simulink model "single_cmg_practice"  (R2023b)
settings: Solver=ode4  StartTime=0.0  StopTime=1000  FixedStep=0.001  RelTol=1e-3
undefined symbols (not defined in the file): As, Cube_L, F_vec, I_rw1, M_c, M_rw, sat, THR_Force, THR_Pos, torque_ext, X, Y, Z
libraries: sm_lib x391, nesl_utility x251, simulink_extras x103, sharedtransform x53, aerolibutil x30, sharedutil x13, simulink x12
(part 13 of 14)

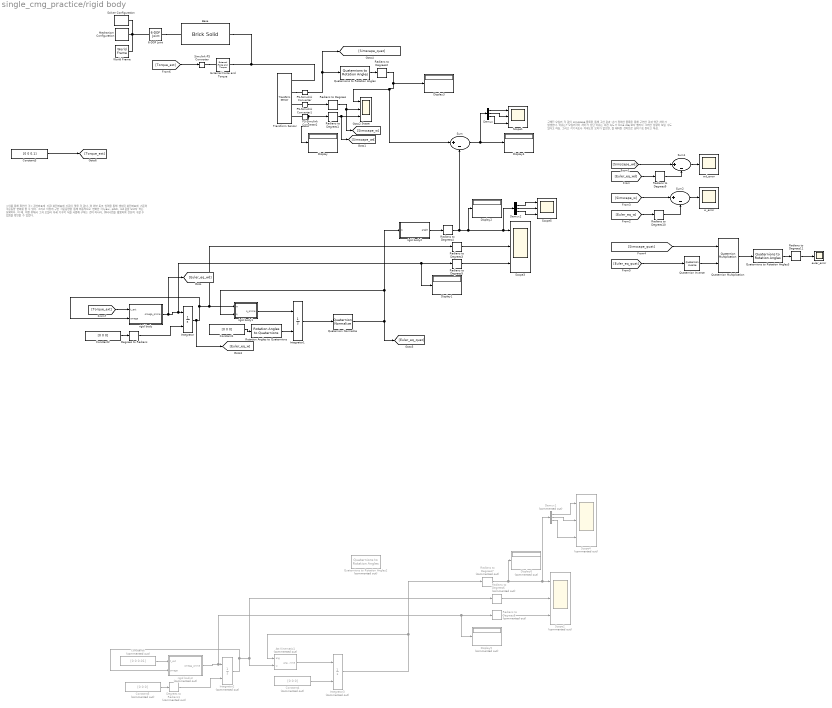
== system single_cmg_practice/rigid body ==
  note: 구해진 오일러 각 값이
      | simscape 블록을 통해 구한 값과 내가 정의한 블록을 통해 구현한 값과
      | 약간 차이가 발생한다.
      | 이유는?
      | 오일러각이 차이가 났던 이유는 회전 속도가 time step보다 빨라서 그러한 상황이 보일 수도 있다고 하심.
      | 그리고 각가속도나 각속도의 오차가 없으면, 잘 제어된 것이므로 넘어가도 된다고 하심.
  note: <이를 통해 확인한 것>
      | 관선좌표계 기준(회전좌표계 기준이 맞을 것 같다.)의 외부 토크 입력을 통해
      | 생성된 회전좌표계 기준의 각운동량 변화를 볼 수 있다.
      |
      | 그리고 이렇게 구한 각운동량을 통해
      | 최종적으로 변화한 각(yaw, pitch, roll)값을 보고자 하는 상황이다.
      | 이 때, 이를 위해서 그저 오일러 자세 기구학 식을 사용해 구하는 것이 아니라,
      | 쿼터니언을 활용하여 간단히 구할 수 있음을 확인할 수 있었다.
  6-DOF Joint : sm_lib/Joints/6-DOF Joint  JointMode=Normal  SenseConstraintForce=off  SenseConstraintForceX=off  SenseConstraintForceY=off  SenseConstraintForceZ=off  SenseConstraintTorque=off  SenseConstraintTorqueX=off  SenseConstraintTorqueY=off  SenseConstraintTorqueZ=off  SenseTotalForce=off  SenseTotalForceX=off  SenseTotalForceY=off  SenseTotalForceZ=off  SenseTotalTorque=off  SenseTotalTorqueX=off  SenseTotalTorqueY=off  SenseTotalTorqueZ=off  CompositeWrenchDir=FollowerOnBase  CompositeWrenchFrame=BaseFrame  PxEquilibriumPosition=0  PxEquilibriumPositionUnits=m  PxSpringStiffness=0  PxSpringStiffnessUnits=N/m  PxDampingCoefficient=0  PxDampingCoefficientUnits=N/(m/s)  PxTorqueActuationMode=NoTorque  PxMotionActuationMode=ComputedMotion  PxSensePosition=off  PxSenseVelocity=off  PxSenseAcceleration=off  PxSenseTorqueForce=off  PxSenseLowerLimitTorqueForce=off  PxSenseUpperLimitTorqueForce=off  PxLowerLimitSpecify=off  PxLowerLimitBound=-1  PxLowerLimitBoundUnits=m  PxLowerLimitStiffness=1e6  PxLowerLimitStiffnessUnits=N/m  PxLowerLimitDamping=1e3  PxLowerLimitDampingUnits=N/(m/s)  PxLowerLimitTransitionRegionWidth=1e-4  PxLowerLimitTransitionRegionWidthUnits=m  PxUpperLimitSpecify=off  PxUpperLimitBound=1  PxUpperLimitBoundUnits=m  PxUpperLimitStiffness=1e6  PxUpperLimitStiffnessUnits=N/m  PxUpperLimitDamping=1e3  PxUpperLimitDampingUnits=N/(m/s)  PxUpperLimitTransitionRegionWidth=1e-4  PxUpperLimitTransitionRegionWidthUnits=m  PxPositionTargetSpecify=off  PxPositionTargetPriority=High  PxPositionTargetValue=0  PxPositionTargetValueUnits=m  PxVelocityTargetSpecify=off  PxVelocityTargetPriority=High  PxVelocityTargetValue=0  PxVelocityTargetValueUnits=m/s  PyEquilibriumPosition=0  PyEquilibriumPositionUnits=m  PySpringStiffness=0  PySpringStiffnessUnits=N/m  PyDampingCoefficient=0  PyDampingCoefficientUnits=N/(m/s)  PyTorqueActuationMode=NoTorque  PyMotionActuationMode=ComputedMotion  PySensePosition=off  PySenseVelocity=off  PySenseAcceleration=off  PySenseTorqueForce=off  PySenseLowerLimitTorqueForce=off  PySenseUpperLimitTorqueForce=off  PyLowerLimitSpecify=off  PyLowerLimitBound=-1  PyLowerLimitBoundUnits=m  PyLowerLimitStiffness=1e6  PyLowerLimitStiffnessUnits=N/m  PyLowerLimitDamping=1e3  PyLowerLimitDampingUnits=N/(m/s)  PyLowerLimitTransitionRegionWidth=1e-4  PyLowerLimitTransitionRegionWidthUnits=m  PyUpperLimitSpecify=off  PyUpperLimitBound=1  PyUpperLimitBoundUnits=m  PyUpperLimitStiffness=1e6  PyUpperLimitStiffnessUnits=N/m  PyUpperLimitDamping=1e3  PyUpperLimitDampingUnits=N/(m/s)  PyUpperLimitTransitionRegionWidth=1e-4  PyUpperLimitTransitionRegionWidthUnits=m  PyPositionTargetSpecify=off  PyPositionTargetPriority=High  PyPositionTargetValue=0  PyPositionTargetValueUnits=m  PyVelocityTargetSpecify=off  PyVelocityTargetPriority=High  PyVelocityTargetValue=0  PyVelocityTargetValueUnits=m/s  PzEquilibriumPosition=0  PzEquilibriumPositionUnits=m  PzSpringStiffness=0  PzSpringStiffnessUnits=N/m  PzDampingCoefficient=0  PzDampingCoefficientUnits=N/(m/s)  PzTorqueActuationMode=NoTorque  PzMotionActuationMode=ComputedMotion  PzSensePosition=off  PzSenseVelocity=off  PzSenseAcceleration=off  PzSenseTorqueForce=off  PzSenseLowerLimitTorqueForce=off  PzSenseUpperLimitTorqueForce=off  PzLowerLimitSpecify=off  PzLowerLimitBound=-1  PzLowerLimitBoundUnits=m  PzLowerLimitStiffness=1e6  PzLowerLimitStiffnessUnits=N/m  PzLowerLimitDamping=1e3  PzLowerLimitDampingUnits=N/(m/s)  PzLowerLimitTransitionRegionWidth=1e-4  PzLowerLimitTransitionRegionWidthUnits=m  PzUpperLimitSpecify=off  PzUpperLimitBound=1  PzUpperLimitBoundUnits=m  PzUpperLimitStiffness=1e6  PzUpperLimitStiffnessUnits=N/m  PzUpperLimitDamping=1e3  PzUpperLimitDampingUnits=N/(m/s)  PzUpperLimitTransitionRegionWidth=1e-4  PzUpperLimitTransitionRegionWidthUnits=m  PzPositionTargetSpecify=off  PzPositionTargetPriority=High  PzPositionTargetValue=0  PzPositionTargetValueUnits=m  PzVelocityTargetSpecify=off  PzVelocityTargetPriority=High  PzVelocityTargetValue=0  PzVelocityTargetValueUnits=m/s  SphEqPosRotationMethod=None  SphEqPosRotationAngleUnits=deg  SphEqPosRotationStandardAxis=+Z  SphEqPosRotationAngle=0.0  SphEqPosRotationArbitraryAxis=[0 0 1]  SphEqPosFollAlignAxisA=+X  SphEqPosBaseAlignAxisA=+Y  SphEqPosFollAlignAxisB=+Y  SphEqPosBaseAlignAxisB=+Z  SphEqPosRotationSequenceAxes=FollowerAxes  SphEqPosRotationSequence=XYX  SphEqPosRotationSequenceAngles=[0 0 0]  SphEqPosRotationSequenceAnglesUnits=deg  SphEqPosRotationMatrix=[1 0 0; 0 1 0; 0 0 1]  SphEqPosQuaternion=[1 0 0 0]  SphSpringStiffness=0  SphSpringStiffnessUnits=N*m/deg  SphDampingCoefficient=0  SphDampingCoefficientUnits=N*m/(deg/s)  SphActuateTorqueX=off  SphActuateTorqueY=off  SphActuateTorqueZ=off  SphActuateTorque=off  SphTorqueActuationMode=NoTorque  SphMotionActuationMode=ComputedMotion  SphActuationFrame=BaseFrame  SphSensePosition=off  SphSenseVelocityX=off  SphSenseVelocityY=off  SphSenseVelocityZ=off  SphSenseVelocity=off  SphSenseAccelerationX=off  SphSenseAccelerationY=off  SphSenseAccelerationZ=off  SphSenseAcceleration=off  SphSenseTorqueX=off  SphSenseTorqueY=off  SphSenseTorqueZ=off  SphSenseTorqueForce=off  SphSenseLowerLimitTorqueMag=off  SphSenseUpperLimitTorqueMag=off  SphSensingFrame=BaseFrame  SphLowerLimitSpecify=off  SphLowerLimitBound=15  SphLowerLimitBoundUnits=deg  SphLowerLimitStiffness=1e4  SphLowerLimitStiffnessUnits=N*m/deg  SphLowerLimitDamping=10  SphLowerLimitDampingUnits=N*m/(deg/s)  SphLowerLimitTransitionRegionWidth=0.1  SphLowerLimitTransitionRegionWidthUnits=deg  SphUpperLimitSpecify=off  SphUpperLimitBound=45  SphUpperLimitBoundUnits=deg  SphUpperLimitStiffness=1e4  SphUpperLimitStiffnessUnits=N*m/deg  SphUpperLimitDamping=10  SphUpperLimitDampingUnits=N*m/(deg/s)  SphUpperLimitTransitionRegionWidth=0.1  SphUpperLimitTransitionRegionWidthUnits=deg  SphPositionTargetRotationMethod=None  SphPositionTargetRotationAngleUnits=deg  SphPositionTargetRotationStandardAxis=+Z  SphPositionTargetRotationAngle=0.0  SphPositionTargetRotationArbitraryAxis=[0 0 1]  SphPositionTargetFollAlignAxisA=+X  SphPositionTargetBaseAlignAxisA=+Y  SphPositionTargetFollAlignAxisB=+Y  SphPositionTargetBaseAlignAxisB=+Z  SphPositionTargetRotationSequenceAxes=FollowerAxes  SphPositionTargetRotationSequence=XYX  SphPositionTargetRotationSequenceAngles=[0 0 0]  SphPositionTargetRotationSequenceAnglesUnits=deg  SphPositionTargetRotationMatrix=[1 0 0; 0 1 0; 0 0 1]  SphPositionTargetQuaternion=[1 0 0 0]  SphPositionTargetSpecify=off  SphPositionTargetPriority=High  SphVelocityTargetValue=[0 0 0]  SphVelocityTargetValueUnits=deg/s  SphVelocityTargetSpecify=off  SphVelocityTargetPriority=High  SphVelocityTargetInFollowerFrame=on
  Att Kinematic1 : MATLAB Function  Commented=on  TreatAsAtomicUnit=on
  Base : sm_lib/Body Elements/Brick Solid  GraphicAmbientColor=[0.15 0.15 0.15 1.0]  BasedOnType=Mass  BrickDimensions=[0.3 0.3 0.3]  BrickDimensionsUnits=m  CenterOfMass=[0 0 0]  CenterOfMassUnits=m  GraphicDiffuseColor=[0.0 0.8 0.8]  Density=1000  DensityUnits=kg/m^3  DoExposeReferenceFrame=on  GraphicEmissiveColor=[0.0 0.0 0.0 1.0]  ExportEntireGeometry=off  SerializedFrames=<Frames><Frame><Id>Frame1</Id><Value><Name>CM_F</Name><Origin><Source>CenterOfMassFrame</Source><FeatureName></FeatureName></Origin><PrimaryAxis><DefinedDirection>+Z</DefinedDirection><Source>ReferenceFrame</Source><SourceDirection>+Z</SourceDirection><FeatureName></FeatureName></PrimaryAxis><SecondaryAxis><DefinedDirection>+X</DefinedDirection><Source>ReferenceFrame</Source><SourceDirection>+X</SourceDirection><FeatureName></FeatureName></SecondaryAxis></Value></Frame></Frames>  MarkerShape=Sphere  MarkerSize=10  GraphicType=FromGeometry  InertiaType=CalculateFromGeometry  Mass=1  MassUnits=kg  MomentsOfInertia=[1 1 1]  MomentsOfInertiaUnits=kg*m^2  GraphicOpacity=1  ProductsOfInertia=[0 0 0]  ProductsOfInertiaUnits=kg*m^2  GraphicShininess=75  GraphicSpecularColor=[0.5 0.5 0.5 1.0]  GraphicVisPropType=SimpleVisualProperties
  Constant1 : Constant  Value=[0 0 0]
  Constant2 : Constant  Value=[0 0 0]
  Constant3 : Constant  Value=[0 0 0.1]
  Constant4 : Constant  Commented=on  Value=[0 0 0]
  Constant5 : Constant  Commented=on  Value=[0 0 0]
  Constant6 : Constant  Commented=on  Value=[0 0 0.01]
  Degrees to Radians : simulink_extras/Transformations/Degrees to Radians
  Degrees to Radians1 : simulink_extras/Transformations/Degrees to Radians  Commented=on
  Demux : Demux  Outputs=3
  Demux1 : Demux  Commented=on  Outputs=3
  Demux2 : Demux  Outputs=3
  Display{,1..4} (5 alike) : Display
  Display5 : Display  Commented=on
  Display6 : Display  Commented=on
  External Force and Torque : sm_lib/Forces and Torques/External Force and Torque  ForceResolutionFrame=AttachedFrame  EnableForceX=off  EnableForceY=off  EnableForceZ=off  EnableForce=off  TorqueResolutionFrame=AttachedFrame  EnableTorqueX=off  EnableTorqueY=off  EnableTorqueZ=off  EnableTorque=on
  Integrator : Integrator  InitialConditionSource=external
  Integrator1 : Integrator  InitialConditionSource=external
  Integrator2 : Integrator  Commented=on  InitialConditionSource=external
  Integrator3 : Integrator  Commented=on  InitialConditionSource=external
  Mechanism Configuration : sm_lib/Utilities/Mechanism Configuration  UniformGravity=None  GravityVector=[0 0 -9.80665]  GravityVectorUnits=m/s^2  LinearizationDelta=0.001  JointModeTransitionNonlinearIterations=2
  PS-Simulink Converter : nesl_utility/PS-Simulink Converter  PhysicalDomain=network_engine_domain  SubClassName=ps_output  LeftPortType=input  RightPortType=output  PseudoPeriodic=off  Frequencies=[]  VectorFormat=inherit  Unit=inherit  AffineConversion=off
  PS-Simulink Converter1 : nesl_utility/PS-Simulink Converter  PhysicalDomain=network_engine_domain  SubClassName=ps_output  LeftPortType=input  RightPortType=output  PseudoPeriodic=off  Frequencies=[]  VectorFormat=inherit  Unit=inherit  AffineConversion=off
  PS-Simulink Converter2 : nesl_utility/PS-Simulink Converter  PhysicalDomain=network_engine_domain  SubClassName=ps_output  LeftPortType=input  RightPortType=output  PseudoPeriodic=off  Frequencies=[]  VectorFormat=inherit  Unit=inherit  AffineConversion=off
  Quaternion Inverse : aerolibutil/Quaternion Inverse
  Quaternion Multiplication : aerolibutil/Quaternion Multiplication
  Quaternion Normalize : sharedutil/Quaternion Normalize  aMode=aMode
  Quaternions to Rotation Angles : sharedtransform/Quaternions to Rotation Angles  rotationOrder=ZYX  aMode=aMode
  Quaternions to Rotation Angles2 : sharedtransform/Quaternions to Rotation Angles  Commented=on  rotationOrder=ZYX  aMode=aMode
  Quaternions to Rotation Angles3 : sharedtransform/Quaternions to Rotation Angles  rotationOrder=ZYX  aMode=aMode
  Radians to Degrees{,1..5,9..11} (9 alike) : simulink_extras/Transformations/Radians to Degrees
  Radians to Degrees6 : simulink_extras/Transformations/Radians to Degrees  Commented=on
  Radians to Degrees7 : simulink_extras/Transformations/Radians to Degrees  Commented=on
  Radians to Degrees8 : simulink_extras/Transformations/Radians to Degrees  Commented=on
  Rotation Angles to Quaternions : sharedtransform/Rotation Angles to Quaternions  rotationOrder=ZYX  aMode=aMode
  Scope{,1,3,5} (4 alike) : Scope  NumInputPorts=3
  Scope2 : Scope  Commented=on  NumInputPorts=3
  Scope4 : Scope  Commented=on  NumInputPorts=3
  Simulink-PS Converter : nesl_utility/Simulink-PS Converter  PhysicalDomain=network_engine_domain  SubClassName=ps_input  LeftPortType=input  RightPortType=output  PseudoPeriodic=off  Frequencies=[]  NoiseDistribution=none  NoiseParameters=[]  Unit=1  AffineConversion=off  FilteringAndDerivatives=provide  SimscapeFilterOrder=1  InputFilterTimeConstant=0.001  UdotUserProvided=0
  Solver Configuration : nesl_utility/Solver Configuration  PhysicalDomain=network_engine_domain  SubClassName=solver  LeftPortType=input  RightPortType=generic  Tones=[]  Harmonics=[]  SimulateNoise=off  Profile=off  UseLocalSampling=off  EnableSwitchedLinearOptims=on  FrequencyDomain=off  UseCCode=off  RelTol=0.001  AbsTol=0.001  MinStep=1e-09  ToWorkspace=off  RevertToSquareIcSolve=off  NumHomotopyIterations=100  PhasorMode=off  PhasorModeNumHarmonics=1  ConsistencySolver=NEWTON_XTOL_AFTER_FTOL  IndexReductionMethod=DerivativeReplacement  DoDC=off  ResidualTolerance=1e-09  ConsistencyTolSource=GLOBAL  ConsistencyAbsTol=0.001  ConsistencyRelTol=0.001  ConsistencyTolFactor=0.001  UseLocalSolver=off  LocalSolverChoice=NE_BACKWARD_EULER_ADVANCER  ResolveIndetEquations=on  FunctionEvalNumThread=1  LocalSolverSampleTime=0.001  DoFixedCost=off  MaxNonlinIter=3  MaxModeIter=2  ComputeImpulses=off  ImpulseIterations=2  LinearAlgebra=auto  LinearAlgebraNumThread=0  EquationFormulation=NE_TIME_EF  DelaysMemoryBudget=1024  AutomaticFiltering=on  FilteringTimeConstant=0.001  PartitionStorageMethod=AS_NEEDED  PartitionMemoryBudget=1024  PartitionMethod=ROBUST  MultibodyUseLocalSolver=off  MultibodyLocalSolverChoice=ODE1  MultibodyLocalSolverSampleTime=0.001
  Sum : Sum  Inputs=|+-
  Sum1 : Sum  Inputs=|+-
  Sum2 : Sum  Inputs=|+-
  Transform Sensor : sm_lib/Frames and Transforms/Transform Sensor  MeasurementFrame=World  RotationSequence=ZYX  SenseAngle=off  SenseAxis=off  SenseQ=on  SenseR=off  SenseRotationSequence=off  SenseOmegaX=off  SenseOmegaY=off  SenseOmegaZ=off  SenseOmega=on  SenseQDot=off  SenseRDot=off  SenseRotationSequenceDot=off  SenseAlphaX=off  SenseAlphaY=off  SenseAlphaZ=off  SenseAlpha=on  SenseQDDot=off  SenseRDDot=off  SenseX=off  SenseY=off  SenseZ=off  SenseXYZ=off  SenseRad=off  SenseAzim=off  SenseDist=off  SenseInc=off  SenseXDot=off  SenseYDot=off  SenseZDot=off  SenseXYZDot=off  SenseRadDot=off  SenseAzimDot=off  SenseDistDot=off  SenseIncDot=off  SenseXDDot=off  SenseYDDot=off  SenseZDDot=off  SenseXYZDDot=off  SenseRadDDot=off  SenseAzimDDot=off  SenseDistDDot=off  SenseIncDDot=off
  World Frame : sm_lib/Frames and Transforms/World Frame
  euler_error : Scope
  rigid body : MATLAB Function  TreatAsAtomicUnit=on
  rigid body1 : MATLAB Function  TreatAsAtomicUnit=on
  rigid body2 : MATLAB Function  TreatAsAtomicUnit=on
  rigid body3 : MATLAB Function  Commented=on  TreatAsAtomicUnit=on
  w_error : Scope
  wd_error : Scope
  wires:
  Radians to Degrees/1 -> [Simscape_w], Scope/2
  Radians to Degrees1/1 -> [Simscape_wd], Scope/3
  PS-Simulink Converter2/1 -> Radians to Degrees1/1, Display/1
  PS-Simulink Converter1/1 -> Radians to Degrees/1
  PS-Simulink Converter/1 -> [Simscape_quat], Quaternions to Rotation Angles/1
  Quaternions to Rotation Angles/1 -> Radians to Degrees2/1
  Quaternion Normalize/1 -> rigid body2/1(q), rigid body1/2(q), [Euler_eq_quat]
  Integrator/1 -> rigid body/2(omega), Radians to Degrees3/1, rigid body1/1(w), [Euler_eq_w]
  Constant1/1 -> Rotation Angles to Quaternions/1
  Rotation Angles to Quaternions/1 -> Integrator1/2
  rigid body1/1(q_prime) -> Integrator1/1
  Integrator1/1 -> Quaternion Normalize/1
  Constant2/1 -> Degrees to Radians/1
  Degrees to Radians/1 -> Integrator/2
  rigid body/1(omega_prime) -> [Euler_eq_wd], Display1/1, Radians to Degrees5/1, Integrator/1
  rigid body2/1(angle) -> Radians to Degrees4/1
  Radians to Degrees3/1 -> Scope3/2
  Radians to Degrees5/1 -> Scope3/3
  Sum/1 -> Demux/1, Display4/1
  Demux/1 -> Scope1/1
  Demux/2 -> Scope1/2
  Demux/3 -> Scope1/3
  Radians to Degrees2/1 -> Sum/1, Scope/1, Display3/1
  Integrator3/1 -> Radians to Degrees7/1, Att Kinematic1/1(ang)
  Radians to Degrees8/1 -> Scope2/3
  Constant4/1 -> Integrator3/2
  rigid body3/1(omega_prime) -> Display5/1, Radians to Degrees8/1, Integrator2/1
  Radians to Degrees6/1 -> Scope2/2
  Radians to Degrees7/1 -> Display6/1, Demux1/1, Scope2/1
  Constant6/1 -> rigid body3/1(t_ext)
  Degrees to Radians1/1 -> Integrator2/2
  Att Kinematic1/1(ang_prime) -> Integrator3/1
  Integrator2/1 -> rigid body3/2(omega), Att Kinematic1/2(w), Radians to Degrees6/1
  Constant5/1 -> Degrees to Radians1/1
  Demux1/2 -> Scope4/2
  Demux1/1 -> Scope4/1
  Demux1/3 -> Scope4/3
  Radians to Degrees4/1 -> Sum/2, Display2/1, Demux2/1, Scope3/1
  Demux2/1 -> Scope5/1
  Demux2/2 -> Scope5/2
  Demux2/3 -> Scope5/3
  Sum1/1 -> wd_error/1
  Sum2/1 -> w_error/1
  [Euler_eq_wd] -> Radians to Degrees9/1
  [Simscape_wd] -> Sum1/1
  Radians to Degrees9/1 -> Sum1/2
  [Euler_eq_w] -> Radians to Degrees10/1
  [Simscape_w] -> Sum2/1
  Radians to Degrees10/1 -> Sum2/2
  [Simscape_quat] -> Quaternion Multiplication/1
  [Euler_eq_quat] -> Quaternion Inverse/1
  Quaternion Inverse/1 -> Quaternion Multiplication/2
  Quaternion Multiplication/1 -> Quaternions to Rotation Angles3/1
  Quaternions to Rotation Angles3/1 -> Radians to Degrees11/1
  Constant3/1 -> [Torque_ext]
  [Torque_ext] -> Simulink-PS Converter/1
  [Torque_ext] -> rigid body/1(t_ext)
  Radians to Degrees11/1 -> euler_error/1
  connections:
  Solver Configuration/RConn1 -- 6-DOF Joint/LConn1 -- Mechanism Configuration/RConn1 -- World Frame/RConn1
  6-DOF Joint/RConn1 -- Base/RConn1
  Base/LConn1 -- External Force and Torque/RConn1 -- Transform Sensor/RConn1
  Transform Sensor/RConn2 -- PS-Simulink Converter/LConn1
  PS-Simulink Converter2/LConn1 -- Transform Sensor/RConn4
  PS-Simulink Converter1/LConn1 -- Transform Sensor/RConn3
  Simulink-PS Converter/RConn1 -- External Force and Torque/LConn1

== system single_cmg_practice/CMG_Gimbal_Angle_Control_Example/Subsystem ==
  angle_cmd : Inport
  angle_mea : Inport  Port=2
  rate_mea : Inport  Port=3
  dt : Inport  Port=4
  Trigger : TriggerPort  TriggerType=either  VariantControl=(inherit)  PortDimensions=1
  Gain : Gain
  Gimbal_Angle_Controller[PID] : MATLAB Function  TreatAsAtomicUnit=on
  t_cmd : Outport
  wires:
  angle_cmd/1 -> Gimbal_Angle_Controller[PID]/1(angle_cmd)
  dt/1 -> Gimbal_Angle_Controller[PID]/4(dt)
  Gimbal_Angle_Controller[PID]/1(t_cmd) -> Gain/1
  angle_mea/1 -> Gimbal_Angle_Controller[PID]/2(angle_mea)
  rate_mea/1 -> Gimbal_Angle_Controller[PID]/3(rate_mea)
  Gain/1 -> t_cmd/1

== matlab function single_cmg_practice/Prac1/rigid body1 ==
  data: w input; q_prime output; q input
function q_prime = fcn(w,q)

F_q = (1/2)*[0 -w(1) -w(2) -w(3);
       w(1) 0 w(3) -w(2);
       w(2) -w(3) 0 w(1);
       w(3) w(2) -w(1) 0];

q_prime = F_q*q;

== matlab function single_cmg_practice/Prac1/rigid body2 ==
  data: angle output; q input
function angle = quat2eulang(q)
% ZYX 회전 가정

% q0 = q(1); q1 = q(2); q2 = q(3); q3 = q(4);
% 
% yaw = atan2(2*(q1*q2 + q0*q3), q0^2+q1^2-q2^2-q3^2);
% 
% s = 2*(q0*q2 - q3*q1);
% s = max(-1, min(1, s));      % clamp
% pitch = asin(s);
% 
% roll = atan2(2*(q2*q3 + q0*q1), q0^2-q1^2-q2^2+q3^2);



% % 'ZYX' 회전에서 DCM을 Body-frame -> 관성좌표계 으로 정의할 때, 각을 구하는 상황.
% % /                cos(psi) cos(theta),                              cos(theta) sin(psi),                   -sin(theta)     \
% % |                                                                                                                         |
% % | cos(psi) sin(phi) sin(theta) - cos(phi) sin(psi), cos(phi) cos(psi) + sin(phi) sin(psi) sin(theta), cos(theta) sin(phi) |
% % |                                                                                                                         |
% % \ sin(phi) sin(psi) + cos(phi) cos(psi) sin(theta), cos(phi) sin(psi) sin(theta) - cos(psi) sin(phi), cos(phi) cos(theta) /
R = quat2DCM(q);
yaw   = atan2(R(1,2), R(1,1));
pitch = -asin(R(1,3));
roll  = atan2(R(2,3), R(3,3));



% angle = [roll, pitch, yaw]';
angle = [yaw, pitch, roll]'; %MATLAB 에서는 [roll, pitch, yaw] 가 아닌 [yaw, pitch, roll] 순으로 값을 반환한다.
% 실제 도움말을 보면, 반환각 벡터에 대해 "Ψ is R1, Θ is R2, and Φ is R3." 으로 나와있는 것을 볼 수 있다.



function R = quat2DCM(q)

q0 = q(1); q1 = q(2); q2 = q(3); q3 = q(4);

%% DCM을 관성좌표계 -> Body-frame 으로 정의할 때의 행렬 
% R = [2*(q0^2 + q1^2)-1, 2*(q1*q2 - q0*q3),2*(q1*q3 + q2*q0);
%      2*(q1*q2 + q0*q3), 2*(q0^2 + q2^2)-1, 2*(q2*q3 - q1*q0);
%      2*(q1*q3 - q2*q0), 2*(q2*q3 + q1*q0), 2*(q0^2 + q3^2)-1];

%% DCM을 Body-frame -> 관성좌표계 으로 정의할 때의 행렬 
R = [q0^2+q1^2-q2^2-q3^2, 2*(q1*q2 + q0*q3), 2*(q1*q3 - q2*q0);
     2*(q1*q2 - q0*q3), q0^2-q1^2+q2^2-q3^2, 2*(q2*q3 + q1*q0);
     2*(q1*q3 + q2*q0), 2*(q2*q3 - q1*q0), q0^2-q1^2-q2^2+q3^2];

end

end

== matlab function single_cmg_practice/Prac1/diff_angle ==
  data: angle_err output; q_err input
function angle_err = calc_diff(q_err)

% normalize
q_err = q_err / norm(q_err);

% safe scalar part
q0 = min(abs(q_err(1)),1);

% angle
angle_err = 2*acos(q0);

end

== matlab function single_cmg_practice/Reaction_Wheel_Simple1/rigid body1 ==
  data: I_rw input; u input; omega_rw_prime output; omega input; omega_rw input
% function omega_rw_prime = fcn(u, omega,omega_rw)
function omega_rw_prime = fcn(I_rw,u, omega,omega_rw)
R=0.015; % Radius([m]) of cylinder(Reaction wheel)
M_rw=0.01; % Mass([kg]) of cylinder(Reaction wheel)
L_rw=0.01; % Length([m]) of cylinder(Reaction wheel)

% % MOI([kg*m^2]) of cylinder(Reaction wheel)
% I_rw=[1/4*M_rw*R^2+1/12*M_rw*L_rw^2 0 0;
%     0 1/4*M_rw*R^2+1/12*M_rw*L_rw^2 0;
%     0 0 1/2*M_rw*R^2];

% omega_rw_prime = inv(I_rw)*(-u - cross(omega,I_rw*omega_rw));
omega_rw_prime = inv(I_rw)*(u - cross(omega,I_rw*omega_rw));
% control intput "u" has same direction with "omega_rw_prime"



% % value1 = inv(I_rw)*(1/2*u - cross(omega,I_rw*omega_rw));
% omega_rw_prime + 3.55271e-15

== matlab function single_cmg_practice/Reaction_Wheel_Simple1/rigid body2 ==
  data: Ib input; t_ext input; omega_prime output; omega input; omega_rw input; omega_rw_prime input
function omega_prime = fcn(Ib, t_ext, omega,omega_rw,omega_rw_prime)
L = [0.3 0.3 0.3]'; %Length([m]) of cube 
M = 10; %Mass([kg]) of cube
% MOI([kg*m^2]) of cube
I = [ 1/12*M*(L(2)^2+L(3)^2) 0 0;
      0 1/12*M*(L(1)^2+L(3)^2) 0;
      0 0 1/12*M*(L(1)^2+L(2)^2)];

R=0.015; % Radius([m]) of cylinder(Reaction wheel)
M_rw=0.01; % Mass([kg]) of cylinder(Reaction wheel)
L_rw=0.01; % Length([m]) of cylinder(Reaction wheel)

% MOI([kg*m^2]) of cylinder(Reaction wheel)
I_rw=[1/4*M_rw*R^2+1/12*M_rw*L_rw^2 0 0;
    0 1/4*M_rw*R^2+1/12*M_rw*L_rw^2 0;
    0 0 1/2*M_rw*R^2];

% Ib=I;


omega_prime = inv(Ib)*(t_ext - I_rw*omega_rw_prime - cross(omega, (Ib*omega) + I_rw*omega_rw));

end

== matlab function single_cmg_practice/Reaction_Wheel_Simple1/deriviation of quaternion2 ==
  data: w input; q_prime output; q input
function q_prime = fcn(w,q)

F_q = (1/2)*[0 -w(1) -w(2) -w(3);
       w(1) 0 w(3) -w(2);
       w(2) -w(3) 0 w(1);
       w(3) w(2) -w(1) 0];

q_prime = F_q*q;

== matlab function single_cmg_practice/Reaction_Wheel_Simple1/quaternion to Euler angle 1 ==
  data: angle output; q input
function angle = quat2eulang(q)
% ZYX 회전 가정

% q0 = q(1); q1 = q(2); q2 = q(3); q3 = q(4);
% 
% yaw = atan2(2*(q1*q2 + q0*q3), q0^2+q1^2-q2^2-q3^2);
% 
% s = 2*(q0*q2 - q3*q1);
% s = max(-1, min(1, s));      % clamp
% pitch = asin(s);
% 
% roll = atan2(2*(q2*q3 + q0*q1), q0^2-q1^2-q2^2+q3^2);



% % 'ZYX' 회전에서 DCM을 Body-frame -> 관성좌표계 으로 정의할 때, 각을 구하는 상황.
% % /                cos(psi) cos(theta),                              cos(theta) sin(psi),                   -sin(theta)     \
% % |                                                                                                                         |
% % | cos(psi) sin(phi) sin(theta) - cos(phi) sin(psi), cos(phi) cos(psi) + sin(phi) sin(psi) sin(theta), cos(theta) sin(phi) |
% % |                                                                                                                         |
% % \ sin(phi) sin(psi) + cos(phi) cos(psi) sin(theta), cos(phi) sin(psi) sin(theta) - cos(psi) sin(phi), cos(phi) cos(theta) /
R = quat2DCM(q);
yaw   = atan2(R(1,2), R(1,1));
pitch = -asin(R(1,3));
roll  = atan2(R(2,3), R(3,3));



% angle = [roll, pitch, yaw]';
angle = [yaw, pitch, roll]'; %MATLAB 에서는 [roll, pitch, yaw] 가 아닌 [yaw, pitch, roll] 순으로 값을 반환한다.
% 실제 도움말을 보면, 반환각 벡터에 대해 "Ψ is R1, Θ is R2, and Φ is R3." 으로 나와있는 것을 볼 수 있다.



function R = quat2DCM(q)

q0 = q(1); q1 = q(2); q2 = q(3); q3 = q(4);

%% DCM을 관성좌표계 -> Body-frame 으로 정의할 때의 행렬 
% R = [2*(q0^2 + q1^2)-1, 2*(q1*q2 - q0*q3),2*(q1*q3 + q2*q0);
%      2*(q1*q2 + q0*q3), 2*(q0^2 + q2^2)-1, 2*(q2*q3 - q1*q0);
%      2*(q1*q3 - q2*q0), 2*(q2*q3 + q1*q0), 2*(q0^2 + q3^2)-1];

%% DCM을 Body-frame -> 관성좌표계 으로 정의할 때의 행렬 
R = [q0^2+q1^2-q2^2-q3^2, 2*(q1*q2 + q0*q3), 2*(q1*q3 - q2*q0);
     2*(q1*q2 - q0*q3), q0^2-q1^2+q2^2-q3^2, 2*(q2*q3 + q1*q0);
     2*(q1*q3 + q2*q0), 2*(q2*q3 - q1*q0), q0^2-q1^2-q2^2+q3^2];

end

end

== matlab function single_cmg_practice/Prac1/deriviation of quaternion2 ==
  data: w input; q_prime output; q input
function q_prime = fcn(w,q)

F_q = (1/2)*[0 -w(1) -w(2) -w(3);
       w(1) 0 w(3) -w(2);
       w(2) -w(3) 0 w(1);
       w(3) w(2) -w(1) 0];

q_prime = F_q*q;

== matlab function single_cmg_practice/Reaction_Wheel_Simple1/deriviation of quaternion1 ==
  data: w input; q_prime output; q input
function q_prime = fcn(w,q)

F_q = (1/2)*[0 -w(1) -w(2) -w(3);
       w(1) 0 w(3) -w(2);
       w(2) -w(3) 0 w(1);
       w(3) w(2) -w(1) 0];

q_prime = F_q*q;

== matlab function single_cmg_practice/Prac1/quaternion to Euler angle 1 ==
  data: angle output; q input
function angle = quat2eulang(q)
% ZYX 회전 가정

% q0 = q(1); q1 = q(2); q2 = q(3); q3 = q(4);
% 
% yaw = atan2(2*(q1*q2 + q0*q3), q0^2+q1^2-q2^2-q3^2);
% 
% s = 2*(q0*q2 - q3*q1);
% s = max(-1, min(1, s));      % clamp
% pitch = asin(s);
% 
% roll = atan2(2*(q2*q3 + q0*q1), q0^2-q1^2-q2^2+q3^2);



% % 'ZYX' 회전에서 DCM을 Body-frame -> 관성좌표계 으로 정의할 때, 각을 구하는 상황.
% % /                cos(psi) cos(theta),                              cos(theta) sin(psi),                   -sin(theta)     \
% % |                                                                                                                         |
% % | cos(psi) sin(phi) sin(theta) - cos(phi) sin(psi), cos(phi) cos(psi) + sin(phi) sin(psi) sin(theta), cos(theta) sin(phi) |
% % |                                                                                                                         |
% % \ sin(phi) sin(psi) + cos(phi) cos(psi) sin(theta), cos(phi) sin(psi) sin(theta) - cos(psi) sin(phi), cos(phi) cos(theta) /
R = quat2DCM(q);
yaw   = atan2(R(1,2), R(1,1));
pitch = -asin(R(1,3));
roll  = atan2(R(2,3), R(3,3));



% angle = [roll, pitch, yaw]';
angle = [yaw, pitch, roll]'; %MATLAB 에서는 [roll, pitch, yaw] 가 아닌 [yaw, pitch, roll] 순으로 값을 반환한다.
% 실제 도움말을 보면, 반환각 벡터에 대해 "Ψ is R1, Θ is R2, and Φ is R3." 으로 나와있는 것을 볼 수 있다.



function R = quat2DCM(q)

q0 = q(1); q1 = q(2); q2 = q(3); q3 = q(4);

%% DCM을 관성좌표계 -> Body-frame 으로 정의할 때의 행렬 
% R = [2*(q0^2 + q1^2)-1, 2*(q1*q2 - q0*q3),2*(q1*q3 + q2*q0);
%      2*(q1*q2 + q0*q3), 2*(q0^2 + q2^2)-1, 2*(q2*q3 - q1*q0);
%      2*(q1*q3 - q2*q0), 2*(q2*q3 + q1*q0), 2*(q0^2 + q3^2)-1];

%% DCM을 Body-frame -> 관성좌표계 으로 정의할 때의 행렬 
R = [q0^2+q1^2-q2^2-q3^2, 2*(q1*q2 + q0*q3), 2*(q1*q3 - q2*q0);
     2*(q1*q2 - q0*q3), q0^2-q1^2+q2^2-q3^2, 2*(q2*q3 + q1*q0);
     2*(q1*q3 + q2*q0), 2*(q2*q3 - q1*q0), q0^2-q1^2-q2^2+q3^2];

end

end

== matlab function single_cmg_practice/Reaction_Wheel_3axis/deriviation of quaternion2 ==
  data: w input; q_prime output; q input
function q_prime = fcn(w,q)

F_q = (1/2)*[0 -w(1) -w(2) -w(3);
       w(1) 0 w(3) -w(2);
       w(2) -w(3) 0 w(1);
       w(3) w(2) -w(1) 0];

q_prime = F_q*q;

== matlab function single_cmg_practice/Prac1/rigid body3 ==
  data: Ib input; t_ext input; omega_prime output; omega input; omega_rw input; omega_rw_prime input; R_rw input; L_rw input; M_rw input
function omega_prime = fcn(Ib, t_ext, omega,omega_rw,omega_rw_prime, R_rw, L_rw, M_rw)
L = [0.3 0.3 0.3]'; %Length([m]) of cube 
M = 10; %Mass([kg]) of cube
% MOI([kg*m^2]) of cube
I = [ 1/12*M*(L(2)^2+L(3)^2) 0 0;
      0 1/12*M*(L(1)^2+L(3)^2) 0;
      0 0 1/12*M*(L(1)^2+L(2)^2)];

% R=0.015; % Radius([m]) of cylinder(Reaction wheel)
% L_rw=0.01; % Length([m]) of cylinder(Reaction wheel)
% M_rw=0.01; % Mass([kg]) of cylinder(Reaction wheel)
R=R_rw;


% MOI([kg*m^2]) of cylinder(Reaction wheel)
I_rw=[1/4*M_rw*R^2+1/12*M_rw*L_rw^2 0 0;
    0 1/4*M_rw*R^2+1/12*M_rw*L_rw^2 0;
    0 0 1/2*M_rw*R^2];

% Ib=I;


omega_prime = inv(Ib)*(t_ext - I_rw*omega_rw_prime - cross(omega, (Ib*omega) + I_rw*omega_rw));

end

== matlab function single_cmg_practice/rigid body/rigid body ==
  data: t_ext input; omega_prime output; omega input
function omega_prime = fcn(t_ext, omega)
L = [0.3 0.3 0.3]'; %Length([m]) of cube 
M = 1; %Mass([kg]) of cube

% Density([kg/m^3]) of cube
density = M/(L(1)*L(2)*L(3));   
% MOI([kg*m^2]) of cube
I = [ 1/12*M*(L(2)^2+L(3)^2) 0 0;
      0 1/12*M*(L(1)^2+L(3)^2) 0;
      0 0 1/12*M*(L(1)^2+L(2)^2)];

omega_prime = inv(I)*(t_ext - cross(omega,I*omega));

== matlab function single_cmg_practice/Reaction_Wheel_3axis/quaternion to Euler angle 1 ==
  data: angle output; q input
function angle = quat2eulang(q)
% ZYX 회전 가정

% q0 = q(1); q1 = q(2); q2 = q(3); q3 = q(4);
% 
% yaw = atan2(2*(q1*q2 + q0*q3), q0^2+q1^2-q2^2-q3^2);
% 
% s = 2*(q0*q2 - q3*q1);
% s = max(-1, min(1, s));      % clamp
% pitch = asin(s);
% 
% roll = atan2(2*(q2*q3 + q0*q1), q0^2-q1^2-q2^2+q3^2);



% % 'ZYX' 회전에서 DCM을 Body-frame -> 관성좌표계 으로 정의할 때, 각을 구하는 상황.
% % /                cos(psi) cos(theta),                              cos(theta) sin(psi),                   -sin(theta)     \
% % |                                                                                                                         |
% % | cos(psi) sin(phi) sin(theta) - cos(phi) sin(psi), cos(phi) cos(psi) + sin(phi) sin(psi) sin(theta), cos(theta) sin(phi) |
% % |                                                                                                                         |
% % \ sin(phi) sin(psi) + cos(phi) cos(psi) sin(theta), cos(phi) sin(psi) sin(theta) - cos(psi) sin(phi), cos(phi) cos(theta) /
R = quat2DCM(q);
yaw   = atan2(R(1,2), R(1,1));
pitch = -asin(R(1,3));
roll  = atan2(R(2,3), R(3,3));



% angle = [roll, pitch, yaw]';
angle = [yaw, pitch, roll]'; %MATLAB 에서는 [roll, pitch, yaw] 가 아닌 [yaw, pitch, roll] 순으로 값을 반환한다.
% 실제 도움말을 보면, 반환각 벡터에 대해 "Ψ is R1, Θ is R2, and Φ is R3." 으로 나와있는 것을 볼 수 있다.



function R = quat2DCM(q)

q0 = q(1); q1 = q(2); q2 = q(3); q3 = q(4);

%% DCM을 관성좌표계 -> Body-frame 으로 정의할 때의 행렬 
% R = [2*(q0^2 + q1^2)-1, 2*(q1*q2 - q0*q3),2*(q1*q3 + q2*q0);
%      2*(q1*q2 + q0*q3), 2*(q0^2 + q2^2)-1, 2*(q2*q3 - q1*q0);
%      2*(q1*q3 - q2*q0), 2*(q2*q3 + q1*q0), 2*(q0^2 + q3^2)-1];

%% DCM을 Body-frame -> 관성좌표계 으로 정의할 때의 행렬 
R = [q0^2+q1^2-q2^2-q3^2, 2*(q1*q2 + q0*q3), 2*(q1*q3 - q2*q0);
     2*(q1*q2 - q0*q3), q0^2-q1^2+q2^2-q3^2, 2*(q2*q3 + q1*q0);
     2*(q1*q3 + q2*q0), 2*(q2*q3 - q1*q0), q0^2-q1^2-q2^2+q3^2];

end

end

== matlab function single_cmg_practice/Reaction_Wheel_Simple3/deriviation of quaternion2 ==
  data: w input; q_prime output; q input
function q_prime = fcn(w,q)

F_q = (1/2)*[0 -w(1) -w(2) -w(3);
       w(1) 0 w(3) -w(2);
       w(2) -w(3) 0 w(1);
       w(3) w(2) -w(1) 0];

q_prime = F_q*q;

== matlab function single_cmg_practice/Reaction_Wheel_Simple3/rigid body2 ==
  data: Wheel_MOI input; Ib input; t_ext input; omega_prime output; omega input; omega_rw input; omega_rw_prime input
function omega_prime = fcn(Wheel_MOI, Ib, t_ext, omega,omega_rw,omega_rw_prime)
% L = [0.3 0.3 0.3]'; %Length([m]) of cube 
% M = 10; %Mass([kg]) of cube
% MOI([kg*m^2]) of cube
% I = [ 1/12*M*(L(2)^2+L(3)^2) 0 0;
%       0 1/12*M*(L(1)^2+L(3)^2) 0;
%       0 0 1/12*M*(L(1)^2+L(2)^2)];

% R=0.015; % Radius([m]) of cylinder(Reaction wheel)
% M_rw=0.01; % Mass([kg]) of cylinder(Reaction wheel)
% L_rw=0.01; % Length([m]) of cylinder(Reaction wheel)

% MOI([kg*m^2]) of cylinder(Reaction wheel)
% I_rw=[1/4*M_rw*R^2+1/12*M_rw*L_rw^2 0 0;
%     0 1/4*M_rw*R^2+1/12*M_rw*L_rw^2 0;
%     0 0 1/2*M_rw*R^2];
% Ib=I;

I_rw3 = Wheel_MOI(3,3);
I_rw = diag([0 0 I_rw3]);

As1 = [0 0 0]';
As2 = [0 0 0]';
As3 = [0 -sind(45) cosd(45)]';

As = [As1, As2, As3];

omega_prime = inv(Ib)*(t_ext - As*I_rw*omega_rw_prime - cross(omega, (Ib*omega) + As*I_rw*omega_rw));

end

== matlab function single_cmg_practice/Reaction_Wheel_3axis/rigid body2 ==
  data: Ib input; t_ext input; omega_prime output; omega input; omega_rw input; omega_rw_prime input; R_rw input; L_rw input; M_rw input
function omega_prime = fcn(Ib, t_ext, omega,omega_rw,omega_rw_prime, R_rw, L_rw, M_rw)
L = [0.3 0.3 0.3]'; %Length([m]) of cube 
M = 10; %Mass([kg]) of cube
% MOI([kg*m^2]) of cube
I = [ 1/12*M*(L(2)^2+L(3)^2) 0 0;
      0 1/12*M*(L(1)^2+L(3)^2) 0;
      0 0 1/12*M*(L(1)^2+L(2)^2)];

% R=0.015; % Radius([m]) of cylinder(Reaction wheel)
% L_rw=0.01; % Length([m]) of cylinder(Reaction wheel)
% M_rw=0.01; % Mass([kg]) of cylinder(Reaction wheel)
R=R_rw;


% MOI([kg*m^2]) of cylinder(Reaction wheel)
I_rw=[1/4*M_rw*R^2+1/12*M_rw*L_rw^2 0 0;
    0 1/4*M_rw*R^2+1/12*M_rw*L_rw^2 0;
    0 0 1/2*M_rw*R^2];

% Ib=I;


omega_prime = inv(Ib)*(t_ext - I_rw*omega_rw_prime - cross(omega, (Ib*omega) + I_rw*omega_rw));

end

== matlab function single_cmg_practice/Reaction_Wheel_Simple2/deriviation of quaternion2 ==
  data: w input; q_prime output; q input
function q_prime = fcn(w,q)

F_q = (1/2)*[0 -w(1) -w(2) -w(3);
       w(1) 0 w(3) -w(2);
       w(2) -w(3) 0 w(1);
       w(3) w(2) -w(1) 0];

q_prime = F_q*q;

== matlab function single_cmg_practice/Single_Reaction_Wheel_PD_Control/deriviation of quaternion2 ==
  data: w input; q_prime output; q input
function q_prime = fcn(w,q)

F_q = (1/2)*[0 -w(1) -w(2) -w(3);
       w(1) 0 w(3) -w(2);
       w(2) -w(3) 0 w(1);
       w(3) w(2) -w(1) 0];

q_prime = F_q*q;

== matlab function single_cmg_practice/Single_Reaction_Wheel_PD_Control/rigid body2 ==
  data: Wheel_MOI input; Ib input; t_ext input; omega_prime output; omega input; omega_rw input; omega_rw_prime input
function omega_prime = fcn(Wheel_MOI, Ib, t_ext, omega,omega_rw,omega_rw_prime)
% L = [0.3 0.3 0.3]'; %Length([m]) of cube 
% M = 10; %Mass([kg]) of cube
% MOI([kg*m^2]) of cube
% I = [ 1/12*M*(L(2)^2+L(3)^2) 0 0;
%       0 1/12*M*(L(1)^2+L(3)^2) 0;
%       0 0 1/12*M*(L(1)^2+L(2)^2)];

% R=0.015; % Radius([m]) of cylinder(Reaction wheel)
% M_rw=0.01; % Mass([kg]) of cylinder(Reaction wheel)
% L_rw=0.01; % Length([m]) of cylinder(Reaction wheel)

% MOI([kg*m^2]) of cylinder(Reaction wheel)
% I_rw=[1/4*M_rw*R^2+1/12*M_rw*L_rw^2 0 0;
%     0 1/4*M_rw*R^2+1/12*M_rw*L_rw^2 0;
%     0 0 1/2*M_rw*R^2];
% Ib=I;

I_rw3 = Wheel_MOI(3,3);
I_rw = diag([0 0 I_rw3]);

As1 = [0 0 0]';
As2 = [0 0 0]';
As3 = [0 -sind(45) cosd(45)]';

As = [As1, As2, As3];

omega_prime = inv(Ib)*(t_ext - As*I_rw*omega_rw_prime - cross(omega, (Ib*omega) + As*I_rw*omega_rw));

end

== matlab function single_cmg_practice/Single_Reaction_Wheel_PD_Control/rigid body1 ==
  data: yaw_err input; w_z_err input; u_cntl output
function u_cntl = fcn(yaw_err, w_z_err)

K1 = 0.0;
K2 = 100.0;

K1 = 0.9;
% K2 = 0.0;

u_cntl = K1*yaw_err + K2*w_z_err;


end

== matlab function single_cmg_practice/CMG_Gimbal_Angle_Control_Example/Subsystem/Gimbal_Angle_Controller[PID] ==
  data: angle_cmd input; angle_mea input; t_cmd output; rate_mea input; dt input
function t_cmd = fcn(angle_cmd, angle_mea, rate_mea, dt)

persistent I_save

if isempty(I_save)
    I_save = 0.0;
end

kp = 1.0;
kd = 2.0;
ki = 0.01;

ang_err = angle_cmd - angle_mea;
rate_err = 0-rate_mea;

t_cmd = kp*ang_err + kd*rate_err + ki*I_save;

I_save = I_save + ang_err*dt;


end

== matlab function single_cmg_practice/Reaction_Wheel_another_Position/deriviation of quaternion2 ==
  data: w input; q_prime output; q input
function q_prime = fcn(w,q)

F_q = (1/2)*[0 -w(1) -w(2) -w(3);
       w(1) 0 w(3) -w(2);
       w(2) -w(3) 0 w(1);
       w(3) w(2) -w(1) 0];

q_prime = F_q*q;

== matlab function single_cmg_practice/Reaction_Wheel_Simple2/rigid body2 ==
  data: Wheel_MOI input; Ib input; t_ext input; omega_prime output; omega input; omega_rw input; omega_rw_prime input
function omega_prime = fcn(Wheel_MOI, Ib, t_ext, omega,omega_rw,omega_rw_prime)
% L = [0.3 0.3 0.3]'; %Length([m]) of cube 
% M = 10; %Mass([kg]) of cube
% MOI([kg*m^2]) of cube
% I = [ 1/12*M*(L(2)^2+L(3)^2) 0 0;
%       0 1/12*M*(L(1)^2+L(3)^2) 0;
%       0 0 1/12*M*(L(1)^2+L(2)^2)];

% R=0.015; % Radius([m]) of cylinder(Reaction wheel)
% M_rw=0.01; % Mass([kg]) of cylinder(Reaction wheel)
% L_rw=0.01; % Length([m]) of cylinder(Reaction wheel)

% MOI([kg*m^2]) of cylinder(Reaction wheel)
% I_rw=[1/4*M_rw*R^2+1/12*M_rw*L_rw^2 0 0;
%     0 1/4*M_rw*R^2+1/12*M_rw*L_rw^2 0;
%     0 0 1/2*M_rw*R^2];
% Ib=I;

I_rw1 = Wheel_MOI(3,3);
I_rw = diag([I_rw1 I_rw1 I_rw1]);

omega_prime = inv(Ib)*(t_ext - I_rw*omega_rw_prime - cross(omega, (Ib*omega) + I_rw*omega_rw));

end

== matlab function single_cmg_practice/Reaction_Wheel_another_Position/rigid body2 ==
  data: Wheel_MOI input; Ib input; t_ext input; omega_prime output; omega input; omega_rw input; omega_rw_prime input
function omega_prime = fcn(Wheel_MOI, Ib, t_ext, omega,omega_rw,omega_rw_prime)

% Ib = diag([0.15, 0.15, 0.15]);
I_rw3 = Wheel_MOI(3,3);
% I_rw3 = 0.001125;

I_rw = diag([0 0 I_rw3]);

As1 = [0 0 0]';
As2 = [0 0 0]';
As3 = [0 -sind(45) cosd(45)]';
% As3 = [0 0 1]';

As = [As1, As2, As3];

omega_prime = inv(Ib)*(t_ext - As*I_rw*omega_rw_prime - cross(omega, (Ib*omega) + As*I_rw*omega_rw));

end

== matlab function single_cmg_practice/Reaction_Wheel_3axis(with 4 wheels)/deriviation of quaternion2 ==
  data: w input; q_prime output; q input
function q_prime = fcn(w,q)

F_q = (1/2)*[0 -w(1) -w(2) -w(3);
       w(1) 0 w(3) -w(2);
       w(2) -w(3) 0 w(1);
       w(3) w(2) -w(1) 0];

q_prime = F_q*q;

== matlab function single_cmg_practice/Reaction_Wheel_3axis(with 4 wheels)/rigid body2 ==
  data: Wheel_MOI input; Ib input; t_ext input; omega_prime output; omega input; omega_rw input; omega_rw_prime input; As input
function omega_prime = fcn(Wheel_MOI, Ib, t_ext, omega,omega_rw,omega_rw_prime, As)

% Reaction wheel MOI Matrix
I_rw1 = Wheel_MOI(3,3);
I_rw2 = Wheel_MOI(3,3);
I_rw3 = Wheel_MOI(3,3);
I_rw4 = Wheel_MOI(3,3);
I_rw = diag([I_rw1 I_rw2 I_rw3 I_rw4]);

omega_prime = inv(Ib)*(t_ext - As*I_rw*omega_rw_prime - cross(omega, (Ib*omega) + As*I_rw*omega_rw));

end

== matlab function single_cmg_practice/Prac1/deriviation of quaternion1 ==
  data: w input; q_prime output; q input
function q_prime = fcn(w,q)

F_q = (1/2)*[0 -w(1) -w(2) -w(3);
       w(1) 0 w(3) -w(2);
       w(2) -w(3) 0 w(1);
       w(3) w(2) -w(1) 0];

q_prime = F_q*q;

== matlab function single_cmg_practice/Prac1/rigid body4 ==
  data: Wheel_MOI input; Ib input; t_ext input; omega_prime output; omega input; omega_rw input; omega_rw_prime input
function omega_prime = fcn(Wheel_MOI, Ib, t_ext, omega,omega_rw,omega_rw_prime)
% L = [0.3 0.3 0.3]'; %Length([m]) of cube 
% M = 10; %Mass([kg]) of cube
% % MOI([kg*m^2]) of cube
% I = [ 1/12*M*(L(2)^2+L(3)^2) 0 0;
%       0 1/12*M*(L(1)^2+L(3)^2) 0;
%       0 0 1/12*M*(L(1)^2+L(2)^2)];

% R=0.015; % Radius([m]) of cylinder(Reaction wheel)
% M_rw=0.01; % Mass([kg]) of cylinder(Reaction wheel)
% L_rw=0.01; % Length([m]) of cylinder(Reaction wheel)

% MOI([kg*m^2]) of cylinder(Reaction wheel)
% I_rw=[1/4*M_rw*R^2+1/12*M_rw*L_rw^2 0 0;
%     0 1/4*M_rw*R^2+1/12*M_rw*L_rw^2 0;
%     0 0 1/2*M_rw*R^2];
% Ib=I;

I_rw1 = Wheel_MOI(3,3);
I_rw = diag([I_rw1 I_rw1 I_rw1]);

omega_prime = inv(Ib)*(t_ext - I_rw*omega_rw_prime - cross(omega, (Ib*omega) + I_rw*omega_rw));

end

== matlab function single_cmg_practice/Thruster_Example_1/Attitude_PD_control ==
  settings: updateMethod=DISCRETE
  data: u_torq output; q_err input; w_err input
function u_torq = att_pd_control(q_err, w_err)

persistent first_flg
persistent I_save

dt = 0.01;

if isempty(first_flg)
    first_flg = 1;
    I_save = [0 0 0]';
end

K1 = 0.1*diag([1 1 1]);
K2 = 0.2*diag([1 1 1]);
K3 = 0.01*diag([1 1 1]);

q_err_ = [q_err(2), q_err(3), q_err(4)]';

u_torq = K1*q_err_ + K2*w_err + K3*I_save;

I_save = I_save + q_err_ * dt;

end

== matlab function single_cmg_practice/Thruster_Example_1/Rigid_Body ==
  data: t_ext input; wd output; w input; F_pwm_mea input; F_vec input; r_thr input
function wd = fcn(t_ext, w, F_pwm_mea, F_vec, r_thr)

Ib = diag([0.015, 0.015, 0.015]);

t_thr = [0 0 0]';
for i=1:12
    Fi = F_pwm_mea(i).*F_vec(:,i);
    Ti = cross(Fi, r_thr(:,i));
    t_thr = t_thr + Ti;
end

wd = inv(Ib)*(t_ext + t_thr - cross(w,Ib*w));

end

== matlab function single_cmg_practice/Reaction_Wheel_3axis(with 4 wheels)/Attitude_PID_control ==
  settings: updateMethod=DISCRETE
  data: u_torq_rw output; q_err input; w_err input; As input
function u_torq_rw = att_pid_control(q_err, w_err, As)
% function u_wd_rw = att_pid_control(q_err, w_err, As, wheel_MOI)

persistent first_flg
persistent I_save

dt = 0.01;

if isempty(first_flg)
    first_flg = 1;
    I_save = [0 0 0]';
end

%input Gain
K1 = 100*0.07*diag([1 1 1]);
K2 = 100*0.07*diag([1 1 1]);
K3 = 1*0.01*diag([1 1 1]);

q_err_ = [q_err(2), q_err(3), q_err(4)]';

u_torq_sat = K1*q_err_ + K2*w_err + K3*I_save;

%torque input
u_torq_rw = (As'*((As*As')\u_torq_sat));
% %Accel input
% u_wd_rw = (As'*((As*As')\u_torq_sat))/wheel_MOI;

I_save = I_save + q_err_ * dt;

% I_save = max(min(I_save, 0.1), -0.1);


end

== matlab function single_cmg_practice/rigid body/rigid body1 ==
  data: w input; q_prime output; q input
function q_prime = fcn(w,q)

F_q = (1/2)*[0 -w(1) -w(2) -w(3);
       w(1) 0 w(3) -w(2);
       w(2) -w(3) 0 w(1);
       w(3) w(2) -w(1) 0];

q_prime = F_q*q;

== matlab function single_cmg_practice/Thruster_Example_1/THR_Allocation ==
  data: pwm output; tau_cmd input; F_on input; f input; r_thr input
function pwm = RCS_Torque2PWM(tau_cmd, F_on, f, r_thr)
%#codegen
% ============================================================
% Minimal RCS allocation: torque command -> PWM duty (0..1)
%   tau ≈ sum_i r_i x (f_i * F_on_i * pwm_i)
%
% Inputs:
%   tau_cmd [3x1]
%   F_on    scalar or [12x1]
%   f       [3x12]  (columns are unit vectors)
%   r_thr   [3x12]  (columns are position vectors wrt CoM)
%
% Output:
%   pwm     [12x1] duty in [0,1]
% ============================================================

% F_on -> 12x1
if isscalar(F_on)
    Fon = F_on * ones(12,1);
else
    Fon = F_on(:);
end

% Build effectiveness matrix B (3x12): tau = B * pwm
B = zeros(3,12);
for i = 1:12
    Fi = Fon(i);
    B(:,i) = cross3(r_thr(:,i), f(:,i) * Fi);  % torque from pwm=1
end

% Unconstrained least-squares solution (minimum-norm)
pwm = B' * ((B*B') \ tau_cmd);

% Clamp to [0,1]
for i=1:12
    if pwm(i) < 0, pwm(i) = 0; end
    if pwm(i) > 1, pwm(i) = 1; end
end

end

function c = cross3(a,b)
c = [ a(2)*b(3) - a(3)*b(2);
      a(3)*b(1) - a(1)*b(3);
      a(1)*b(2) - a(2)*b(1) ];
end

== matlab function single_cmg_practice/Thruster_Example_1/Quaternion_Kinematics ==
  data: w input; qd output; q input
function qd = fcn(w,q)

F_q = (1/2)*[0 -w(1) -w(2) -w(3);
       w(1) 0 w(3) -w(2);
       w(2) -w(3) 0 w(1);
       w(3) w(2) -w(1) 0];

qd = F_q*q;

end

== matlab function single_cmg_practice/rigid body/rigid body2 ==
  data: angle output; q input
function angle = quat2eulang(q)
% ZYX 회전 가정

% q0 = q(1); q1 = q(2); q2 = q(3); q3 = q(4);
% 
% yaw = atan2(2*(q1*q2 + q0*q3), q0^2+q1^2-q2^2-q3^2);
% 
% s = 2*(q0*q2 - q3*q1);
% s = max(-1, min(1, s));      % clamp
% pitch = asin(s);
% 
% roll = atan2(2*(q2*q3 + q0*q1), q0^2-q1^2-q2^2+q3^2);



% % 'ZYX' 회전에서 DCM을 Body-frame -> 관성좌표계 으로 정의할 때, 각을 구하는 상황.
% % /                cos(psi) cos(theta),                              cos(theta) sin(psi),                   -sin(theta)     \
% % |                                                                                                                         |
% % | cos(psi) sin(phi) sin(theta) - cos(phi) sin(psi), cos(phi) cos(psi) + sin(phi) sin(psi) sin(theta), cos(theta) sin(phi) |
% % |                                                                                                                         |
% % \ sin(phi) sin(psi) + cos(phi) cos(psi) sin(theta), cos(phi) sin(psi) sin(theta) - cos(psi) sin(phi), cos(phi) cos(theta) /
R = quat2DCM(q);
yaw   = atan2(R(1,2), R(1,1));
pitch = -asin(R(1,3));
roll  = atan2(R(2,3), R(3,3));



% angle = [roll, pitch, yaw]';
angle = [yaw, pitch, roll]'; %MATLAB 에서는 [roll, pitch, yaw] 가 아닌 [yaw, pitch, roll] 순으로 값을 반환한다.
% 실제 도움말을 보면, 반환각 벡터에 대해 "Ψ is R1, Θ is R2, and Φ is R3." 으로 나와있는 것을 볼 수 있다.



function R = quat2DCM(q)

q0 = q(1); q1 = q(2); q2 = q(3); q3 = q(4);

%% DCM을 관성좌표계 -> Body-frame 으로 정의할 때의 행렬 
% R = [2*(q0^2 + q1^2)-1, 2*(q1*q2 - q0*q3),2*(q1*q3 + q2*q0);
%      2*(q1*q2 + q0*q3), 2*(q0^2 + q2^2)-1, 2*(q2*q3 - q1*q0);
%      2*(q1*q3 - q2*q0), 2*(q2*q3 + q1*q0), 2*(q0^2 + q3^2)-1];

%% DCM을 Body-frame -> 관성좌표계 으로 정의할 때의 행렬 
R = [q0^2+q1^2-q2^2-q3^2, 2*(q1*q2 + q0*q3), 2*(q1*q3 - q2*q0);
     2*(q1*q2 - q0*q3), q0^2-q1^2+q2^2-q3^2, 2*(q2*q3 + q1*q0);
     2*(q1*q3 + q2*q0), 2*(q2*q3 - q1*q0), q0^2-q1^2-q2^2+q3^2];

end

end

== matlab function single_cmg_practice/Reaction_Wheel_Simple1/rigid body ==
  data: t_ext input; omega_prime output; omega input; omega_rw input; omega_rw_prime input
% function omega_prime = fcn(t_ext, omega,u)
function omega_prime = fcn(t_ext, omega,omega_rw,omega_rw_prime)
% function omega_prime = fcn(Ib,t_ext, omega,omega_rw,omega_rw_prime)
L = [0.3 0.3 0.3]'; %Length([m]) of cube 
M = 10; %Mass([kg]) of cube

R=0.015; % Radius([m]) of cylinder(Reaction wheel)
M_rw=0.01; % Mass([kg]) of cylinder(Reaction wheel)
L_rw=0.01; % Length([m]) of cylinder(Reaction wheel)

% Density([kg/m^3]) of cube
density = M/(L(1)*L(2)*L(3));   
% MOI([kg*m^2]) of cube
I = [ 1/12*M*(L(2)^2+L(3)^2) 0 0;
      0 1/12*M*(L(1)^2+L(3)^2) 0;
      0 0 1/12*M*(L(1)^2+L(2)^2)];

% MOI([kg*m^2]) of cylinder(Reaction wheel)
I_rw=[1/4*M_rw*R^2+1/12*M_rw*L_rw^2 0 0;
    0 1/4*M_rw*R^2+1/12*M_rw*L_rw^2 0;
    0 0 1/2*M_rw*R^2];

Ib = I; % body's MOI should include whole MOI.
        % No!! Ib is just cube's MOI!!

%control input torque
% u=-(I_rw*omega_rw_prime+cross(omega,I_rw*omega_rw));
u=I_rw*omega_rw_prime+cross(omega,I_rw*omega_rw);

% omega_prime = inv(Ib)*(t_ext+u - cross(omega,Ib*omega));
omega_prime = inv(Ib)*(t_ext-u - cross(omega,Ib*omega));
% control intput "u" has opposite direction with "t_ext"

== matlab function single_cmg_practice/rigid body/Att Kinematic1 ==
  data: ang input; w input; ang_prime output
function ang_prime = fcn(ang,w)

phi = ang(1);   %roll
theta = ang(2); %pitch
psi = ang(3);   %yaw

Att = [1 sin(phi)*tan(theta) cos(phi)*tan(theta);
    0 cos(phi) -sin(phi);
    0 sin(phi)*sec(theta) cos(phi)*sec(theta)];

ang_prime = Att*w;

== matlab function single_cmg_practice/rigid body/rigid body3 ==
  data: t_ext input; omega_prime output; omega input
function omega_prime = fcn(t_ext, omega)
L = [0.3 0.3 0.3]'; %Length([m]) of cube 
M = 1; %Mass([kg]) of cube

% Density([kg/m^3]) of cube
density = M/(L(1)*L(2)*L(3));   
% MOI([kg*m^2]) of cube
I = [ 1/12*M*(L(2)^2+L(3)^2) 0 0;
    0 1/12*M*(L(1)^2+L(3)^2) 0;
    0 0 1/12*M*(L(1)^2+L(2)^2)];

omega_prime = inv(I)*(t_ext - cross(omega,I*omega));

== matlab function single_cmg_practice/Reaction_Wheel_Simple1/deriviation of quaternion ==
  data: w input; q_prime output; q input
function q_prime = fcn(w,q)

F_q = (1/2)*[0 -w(1) -w(2) -w(3);
       w(1) 0 w(3) -w(2);
       w(2) -w(3) 0 w(1);
       w(3) w(2) -w(1) 0];

q_prime = F_q*q;
